simulink model "ADCS_onOrbit"  (R2024b)
settings: Solver=ode4  StartTime=0.0  StopTime=tspan  FixedStep=baseRate  RelTol=1e-3
values from neighbouring files (symbols this model uses):
  A_list = [10*30; 10*30; 10*10; 10*30; 10*30; 10*10] * 1e-04    [adcsInitializer.m]
  A_m = eye(3)    [adcsInitializer.m]
  A_w = eye(3)    [adcsInitializer.m]
  CD = 2.3    [adcsInitializer.m]
  COP = [xAxis/2   0          0 ... (first row only)    [adcsInitializer.m]
  dt = 1    [adcsInitializer.m]
  dYear = decyear(YYYY,MM,DD)    [adcsInitializer.m]
  eta = 0.3    [adcsInitializer.m]
  J_body = [ I_xx  I_xy  I_xz ... (first row only)    [adcsInitializer.m]
  JD0 = juliandate(YYYY,MM,DD,HH,MIN,SEC)    [adcsInitializer.m]
  m = 4    [adcsInitializer.m]
  mag_moment = [0.005; 0.005; 0.005]    [adcsInitializer.m]
  mode = mode(:)    [generateOutput.m]
  mu = 398600.4418    [adcsInitializer.m]    (also in montecarlo.m = mean(W,2))
  n_list = [1 0 0; 0 1 0; 0 0 1; -1 0 0; 0 -1 0; 0 0 -1]    [adcsInitializer.m]
  p = 0.00000451    (= 4.51e-06)    [adcsInitializer.m]
  R = blkdiag(sigma_S^2*eye(3), sigma_B^2*eye(3))    [adcsInitializer.m]
  rE = 6378.14    [adcsInitializer.m]
  sigma_b = deg2rad(0.04)/3600    [adcsInitializer.m]
  sigma_B = 0.001    [adcsInitializer.m]
  sigma_g = deg2rad(0.1)/sqrt(3600)    [adcsInitializer.m]
  sigma_S = deg2rad(0.01)    [adcsInitializer.m]
  T = 1    [adcsInitializer.m]
  wE = [0 0 15.04*(pi/180)*(1/3600)]    [adcsInitializer.m]
  wW_1 = 0    [adcsInitializer.m]
  wW_2 = 0    [adcsInitializer.m]
  wW_3 = 0    [adcsInitializer.m]
undefined symbols (not defined in the file or in its folder): DiscIntNeverNeededParam, J_wheels, K_d, K_p, K_w, n, period, q1_ini, q2_ini, q3_ini, q4_ini, r_I_ini, truevals, useFilter, v_I_ini, wB_1, wB_2, wB_3
libraries: simulink_extras x15, matrix_library x3
(part 1 of 2)
settings Model: Creator=nimis  LastModifiedBy=nimis
settings DebuggingCC: AlgebraicLoopMsg=none

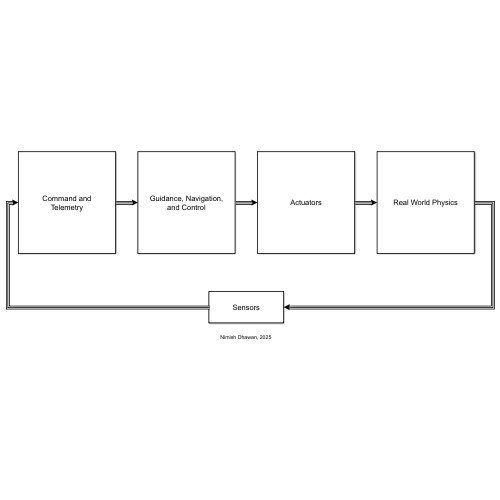
[thumbnail: Simulink's stored preview of the top-level diagram]
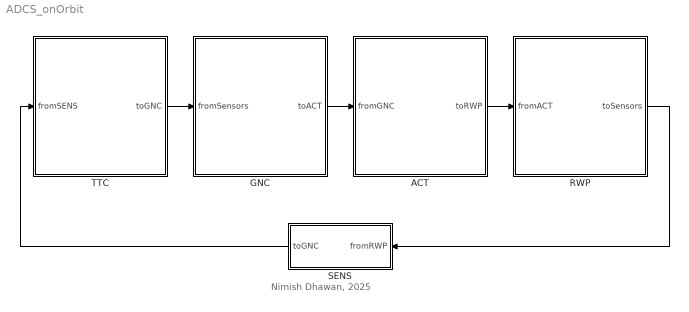
== system ADCS_onOrbit ==
  note: Nimish Dhawan, 2025
  ACT : Subsystem
      mask Display: disp('Actuators');
  GNC : Subsystem
      mask Display: disp('Guidance, Navigation,\nand Control');
  RWP : Subsystem
      mask Display: disp('Real World Physics');
  SENS : Subsystem
      mask Display: disp('Sensors');
  TTC : Subsystem
      mask Display: disp('Command and\nTelemetry');
  wires:
  SENS/1(toGNC) -> TTC/1(fromSENS)
  TTC/1(toGNC) -> GNC/1(fromSensors)
  GNC/1(toACT) -> ACT/1(fromGNC)
  RWP/1(toSensors) -> SENS/1(fromRWP)
  ACT/1(toRWP) -> RWP/1(fromACT)

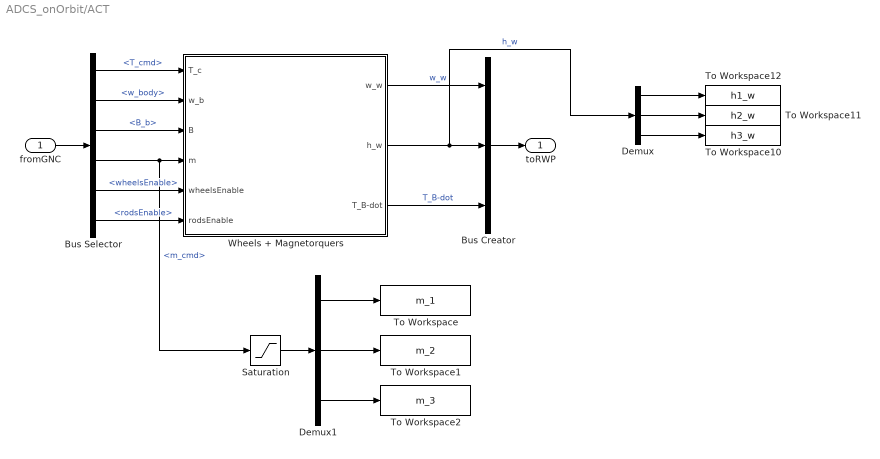
== system ADCS_onOrbit/ACT ==
  fromGNC : Inport
  Bus Creator : BusCreator  Inputs=3
  Bus Selector : BusSelector  OutputSignals=T_cmd,w_body,B_b,m_cmd,wheelsEnable,rodsEnable
  Demux : Demux  Outputs=3
  Demux1 : Demux  Outputs=3
  Saturation : Saturate  UpperLimit=0.2  LowerLimit=-0.2
  To Workspace : ToWorkspace  VariableName=m_1  SampleTime=-1
  To Workspace1 : ToWorkspace  VariableName=m_2  SampleTime=-1
  To Workspace10 : ToWorkspace  VariableName=h3_w  SampleTime=-1
      settings: Save2DSignal=2-D array (concatenate along first dimension)
  To Workspace11 : ToWorkspace  VariableName=h2_w  SampleTime=-1
      settings: Save2DSignal=2-D array (concatenate along first dimension)
  To Workspace12 : ToWorkspace  VariableName=h1_w  SampleTime=-1
      settings: Save2DSignal=2-D array (concatenate along first dimension)
  To Workspace2 : ToWorkspace  VariableName=m_3  SampleTime=-1
  Wheels + Magnetorquers : Subsystem
      mask Display: disp('Wheels + Magnetorquers');
  toRWP : Outport
  wires:
  Bus Selector/2 -> Wheels + Magnetorquers/2(w_b)  "<w_body>"
  Bus Selector/3 -> Wheels + Magnetorquers/3(B)  "<B_b>"
  Bus Selector/4 -> Wheels + Magnetorquers/4(m), Saturation/1  "<m_cmd>"
  Wheels + Magnetorquers/3(T_B-dot) -> Bus Creator/3  "T_B-dot"
  Demux/3 -> To Workspace10/1
  Demux/2 -> To Workspace11/1
  Wheels + Magnetorquers/2(h_w) -> Demux/1, Bus Creator/2  "h_w"
  Demux/1 -> To Workspace12/1
  Demux1/1 -> To Workspace/1
  Saturation/1 -> Demux1/1
  Demux1/2 -> To Workspace1/1
  Demux1/3 -> To Workspace2/1
  fromGNC/1 -> Bus Selector/1
  Bus Selector/1 -> Wheels + Magnetorquers/1(T_c)  "<T_cmd>"
  Bus Creator/1 -> toRWP/1
  Wheels + Magnetorquers/1(w_w) -> Bus Creator/1  "w_w"
  Bus Selector/5 -> Wheels + Magnetorquers/5(wheelsEnable)  "<wheelsEnable>"
  Bus Selector/6 -> Wheels + Magnetorquers/6(rodsEnable)  "<rodsEnable>"

== system ADCS_onOrbit/GNC ==
  fromSensors : Inport
  Bus Creator : BusCreator  Inputs=7
  Bus Selector : BusSelector  OutputSignals=fromSENS,opMode
  Bus Selector1 : BusSelector  OutputSignals=fromSENS.state_act,fromSENS.s_I,opMode
  Bus Selector2 : BusSelector  OutputSignals=fromSENS.h_w,opMode,wheelsEnable,rodsEnable
  Control : Subsystem
  Guidance : Subsystem
      settings: PortSchema="{\"entries\":[{\"content\":{\"sides\":[{\"content\":{},\"type\":\"ConnectorPlacement.EquallySpacedRectSide\",\"uuid\":\"1b864df5-58d8-4c90-91c9-86121554aa4c\"},{\"content\":{\"side\":\"RIGHT\"},\"type\":\"ConnectorPlacement.EquallySpacedRectSide\",\"uuid\":\"8c8748bb-fc8a-40e3-a181-470f6593a9be\"},{\"content\":{\"connectorIds\":[\"Out1\"],\"side\":\"TOP\"},\"type\":\"ConnectorPlacement.EquallySpacedRectSide\",\"uuid\":\"61030da7-ff27-4452-a972-ecb51c641993\"},{\"content\":{\"connectorIds\":[\"In1\",\"In2\",\"In3\",\"In4\",\"In5\"],\"side\":\"BOTTOM\"},\"type\":\"ConnectorPlacement.EquallySpacedRectSide\",\"uuid\":\"02e92b40-894b-4184-ac6b-030597657a3a\"}]},\"type\":\"ConnectorPlacement.EquallySpacedConnector\",\"uuid\":\"ef994289-427e-4085-aff4-2d7817af2aa7\"}],\"packageUris\":[\"http://schema.mathworks.com/mf0/Connector/R2020b\"],\"version\":\"1.0\"}"
  Navigation : Subsystem
  toACT : Outport
  wires:
  Control/4(m) -> Bus Creator/4  "m_cmd"
  Control/2(B_b) -> Bus Creator/2  "B_b"
  Control/1(T_c) -> Bus Creator/1  "T_cmd"
  Bus Selector2/1 -> Control/4(h_w)  "<h_w>"
  Control/3(w_b) -> Bus Creator/3  "w_body"
  fromSensors/1 -> Bus Selector1/1, Bus Selector2/1, Bus Selector/1
  Bus Creator/1 -> toACT/1
  Navigation/1(w_est) -> Control/2(w_body), Guidance/4(w_est)
  Navigation/2(q_est) -> Guidance/5(q_est)  "q_est"
  Navigation/3(B_est) -> Control/3(B)
  Bus Selector1/1 -> Guidance/1(state)  "<state_act>"
  Bus Selector1/2 -> Guidance/2(s_I)  "<s_I>"
  Bus Selector1/3 -> Guidance/3(opMode)  "<opMode>"
  Bus Selector/1 -> Navigation/1(fromSENS)  "<fromSENS>"
  Bus Selector2/2 -> Control/5(opMode), Bus Creator/5  "<opMode>"
  Bus Selector/2 -> Navigation/2(opMode)  "<opMode>"
  Bus Selector2/3 -> Bus Creator/6  "<wheelsEnable>"
  Bus Selector2/4 -> Bus Creator/7  "<rodsEnable>"
  Guidance/1(error) -> Control/1(error)

== system ADCS_onOrbit/RWP ==
  fromACT : Inport
  Environment : Subsystem
  Nonlinear Spacecraft : Subsystem
  Orbit Propator : Subsystem
  Subsystem : Subsystem
  toSensors : Outport
  wires:
  Orbit Propator/1(propOut) -> Environment/1(propIn)
  fromACT/1 -> Nonlinear Spacecraft/2(fromACT)
  Environment/1(envOut) -> Nonlinear Spacecraft/1(T_ext)
  Nonlinear Spacecraft/1(scOut) -> Subsystem/1(fromSC), Orbit Propator/1(q_sc)
  Subsystem/1(RWPoutput) -> toSensors/1

== system ADCS_onOrbit/SENS ==
  fromRWP : Inport
  Bus Creator : BusCreator  Inputs=10
  Bus Selector : BusSelector  OutputSignals=state,B_b,s_B,w_sc
  Bus Selector1 : BusSelector  OutputSignals=h_w,r_SI,q_sc
  Bus Selector2 : BusSelector  OutputSignals=B_I,s_I,T_ext
  GPS : Subsystem
  Gyroscope : Subsystem
  Magnetometer : Subsystem
  Sun Sensor : Subsystem
  toGNC : Outport
  wires:
  fromRWP/1 -> Bus Selector2/1, Bus Selector1/1, Bus Selector/1
  Bus Selector/1 -> GPS/1(state)  "<state>"
  GPS/1(state_act) -> Bus Creator/1  "state_act"
  Bus Selector/2 -> Magnetometer/1(B_b)  "<B_b>"
  Magnetometer/1(B_meas) -> Bus Creator/2  "B_b_meas"
  Bus Selector/3 -> Sun Sensor/1(s_B)  "<s_B>"
  Sun Sensor/1(s_B_meas) -> Bus Creator/3  "s_B_meas"
  Bus Creator/1 -> toGNC/1
  Bus Selector/4 -> Gyroscope/1(w_sc)  "<w_sc>"
  Gyroscope/1(w_meas) -> Bus Creator/4  "w_sc_meas"
  Bus Selector1/3 -> Bus Creator/7  "<q_sc>"
  Bus Selector1/2 -> Bus Creator/6  "<r_SI>"
  Bus Selector1/1 -> Bus Creator/5  "<h_w>"
  Bus Selector2/2 -> Bus Creator/9  "<s_I>"
  Bus Selector2/1 -> Bus Creator/8  "<B_I>"
  Bus Selector2/3 -> Bus Creator/10  "<T_ext>"

== system ADCS_onOrbit/TTC ==
  fromSENS : Inport
  Bus Creator : BusCreator  Inputs=4
  Clock : Clock
  Constant : Constant  Value=mode
  From Spreadsheet : FromSpreadsheet  FileName=controlCommand.xlsx  SheetName=commands  Range=B1:E1000  InterpolationWithinTimeRange=Zero order hold  ExtrapolationAfterLastDataPoint=Hold last value
  MATLAB Function : MATLAB Function  TreatAsAtomicUnit=on
  Mux : Mux  Inputs=3
  RES : Subsystem
      mask Display: disp('Telemetry');
  toGNC : Outport
  tag scope: simTime=global
  wires:
  fromSENS/1 -> Bus Creator/1  "fromSENS"
  Bus Creator/1 -> toGNC/1
  Constant/1 -> MATLAB Function/1(internal)
  From Spreadsheet/1 -> Mux/1  "modeData"
  MATLAB Function/1(mode) -> Bus Creator/2  "opMode"
  From Spreadsheet/3 -> Mux/3  "wheelsData"
  From Spreadsheet/2 -> Mux/2  "rodsData"
  Mux/1 -> MATLAB Function/2(fromTable)
  MATLAB Function/2(wheelsEnable) -> Bus Creator/3  "wheelsEnable"
  MATLAB Function/3(rodsEnable) -> Bus Creator/4  "rodsEnable"
  Clock/1 -> [simTime]

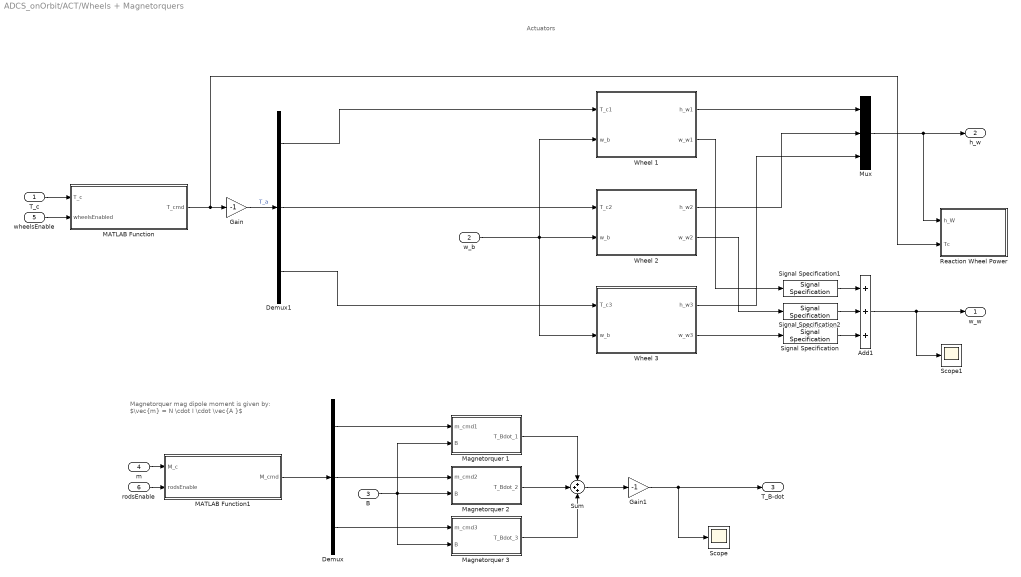
== system ADCS_onOrbit/ACT/Wheels + Magnetorquers ==
  note: Actuators
  note: Magnetorquer mag dipole moment is given by:
      | $\vec{m} = N \cdot I \cdot \vec{A }$
  T_c : Inport
  w_b : Inport  Port=2
  B : Inport  Port=3
  m : Inport  Port=4
  wheelsEnable : Inport  Port=5
  rodsEnable : Inport  Port=6
  Add1 : Sum  Inputs=+++
  Demux : Demux  Outputs=3
  Demux1 : Demux  Outputs=3
  Gain : Gain  Gain=-1
  Gain1 : Gain  Gain=-1
  MATLAB Function : MATLAB Function  TreatAsAtomicUnit=on
  MATLAB Function1 : MATLAB Function  TreatAsAtomicUnit=on
  Magnetorquer 1 : Subsystem
  Magnetorquer 2 : Subsystem
  Magnetorquer 3 : Subsystem
  Mux : Mux  Inputs=3
  Reaction Wheel Power : Subsystem
  Scope : Scope
  Scope1 : Scope
  Signal Specification : SignalSpecification  Dimensions=[3,1]
  Signal Specification1 : SignalSpecification  Dimensions=[3,1]
  Signal Specification2 : SignalSpecification  Dimensions=[3,1]
  Sum : Sum  Inputs=+++
  Wheel 1 : Subsystem
  Wheel 2 : Subsystem
  Wheel 3 : Subsystem
  w_w : Outport
  h_w : Outport  Port=2
  T_B-dot : Outport  Port=3
  wires:
  Gain/1 -> Demux1/1  "T_a"
  T_c/1 -> MATLAB Function/1(T_c)
  Demux1/1 -> Wheel 1/1(T_c1)
  Wheel 3/1(h_w3) -> Mux/3
  Wheel 1/2(w_w1) -> Signal Specification1/1
  w_b/1 -> Wheel 3/2(w_b), Wheel 2/2(w_b), Wheel 1/2(w_b)
  Demux1/2 -> Wheel 2/1(T_c2)
  Mux/1 -> Reaction Wheel Power/1(h_W), h_w/1
  Wheel 1/1(h_w1) -> Mux/1
  Wheel 3/2(w_w3) -> Signal Specification/1
  Demux1/3 -> Wheel 3/1(T_c3)
  Wheel 2/2(w_w2) -> Signal Specification2/1
  Gain1/1 -> T_B-dot/1, Scope/1
  Magnetorquer 3/1(T_Bdot_3) -> Sum/3
  Demux/2 -> Magnetorquer 2/1(m_cmd2)
  Magnetorquer 2/1(T_Bdot_2) -> Sum/2
  Demux/3 -> Magnetorquer 3/1(m_cmd3)
  Sum/1 -> Gain1/1
  Magnetorquer 1/1(T_Bdot_1) -> Sum/1
  B/1 -> Magnetorquer 2/2(B), Magnetorquer 3/2(B), Magnetorquer 1/2(B)
  Demux/1 -> Magnetorquer 1/1(m_cmd1)
  m/1 -> MATLAB Function1/1(M_c)
  Wheel 2/1(h_w2) -> Mux/2
  wheelsEnable/1 -> MATLAB Function/2(wheelsEnabled)
  rodsEnable/1 -> MATLAB Function1/2(rodsEnable)
  MATLAB Function1/1(M_cmd) -> Demux/1
  MATLAB Function/1(T_cmd) -> Reaction Wheel Power/2(Tc), Gain/1
  Add1/1 -> Scope1/1, w_w/1
  Signal Specification/1 -> Add1/3
  Signal Specification1/1 -> Add1/1
  Signal Specification2/1 -> Add1/2

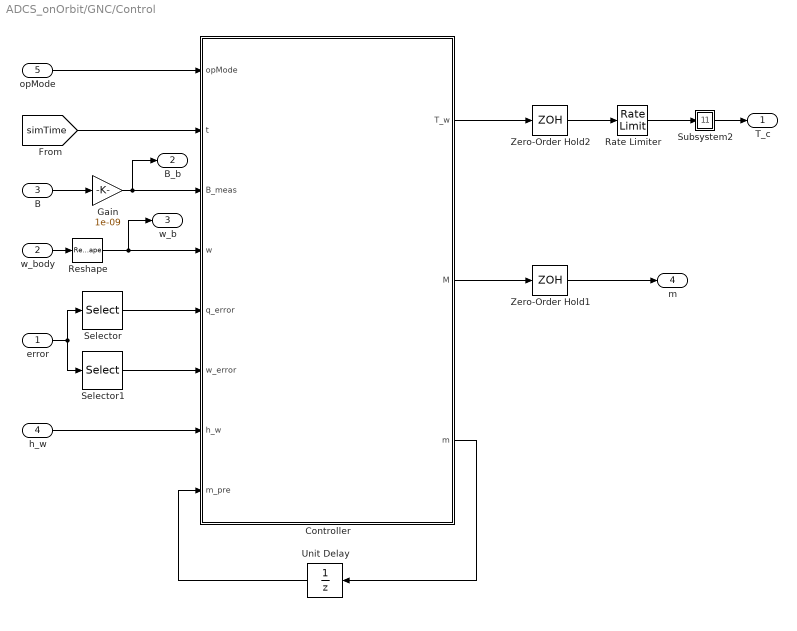
== system ADCS_onOrbit/GNC/Control ==
  error : Inport
  w_body : Inport  Port=2
  B : Inport  Port=3
  h_w : Inport  Port=4
  opMode : Inport  Port=5
  Controller : MATLAB Function  TreatAsAtomicUnit=on
  Gain : Gain  Gain=1e-09
  Rate Limiter : RateLimiter  RisingSlewLimit=5e-07  FallingSlewLimit=-5e-07  SampleTimeMode=inherited
  Reshape : Reshape  OutputDimensionality=Column vector (2-D)  OutputDimensions=[3,1]
  Selector : Selector  InputPortWidth=7  IndexOptions=Index vector (dialog)  Indices=[4 5 6 7]  OutputSizes=1
  Selector1 : Selector  InputPortWidth=7  IndexOptions=Index vector (dialog)  Indices=[1 2 3]  OutputSizes=1
  Subsystem2 : Subsystem
  Unit Delay : UnitDelay  SampleTime=-1  HasFrameUpgradeWarning=on
  Zero-Order Hold1 : ZeroOrderHold  SampleTime=-1
  Zero-Order Hold2 : ZeroOrderHold  SampleTime=-1
  T_c : Outport
  B_b : Outport  Port=2
  w_b : Outport  Port=3
  m : Outport  Port=4
  wires:
  Reshape/1 -> w_b/1, Controller/4(w)
  Gain/1 -> B_b/1, Controller/3(B_meas)
  Controller/1(T_w) -> Zero-Order Hold2/1
  B/1 -> Gain/1
  Zero-Order Hold1/1 -> m/1
  error/1 -> Selector/1, Selector1/1
  Subsystem2/1(T_c) -> T_c/1
  opMode/1 -> Controller/1(opMode)
  [simTime] -> Controller/2(t)
  Selector/1 -> Controller/5(q_error)
  Selector1/1 -> Controller/6(w_error)
  w_body/1 -> Reshape/1
  h_w/1 -> Controller/7(h_w)
  Controller/2(M) -> Zero-Order Hold1/1
  Zero-Order Hold2/1 -> Rate Limiter/1
  Controller/3(m) -> Unit Delay/1
  Unit Delay/1 -> Controller/8(m_pre)
  Rate Limiter/1 -> Subsystem2/1(In1)

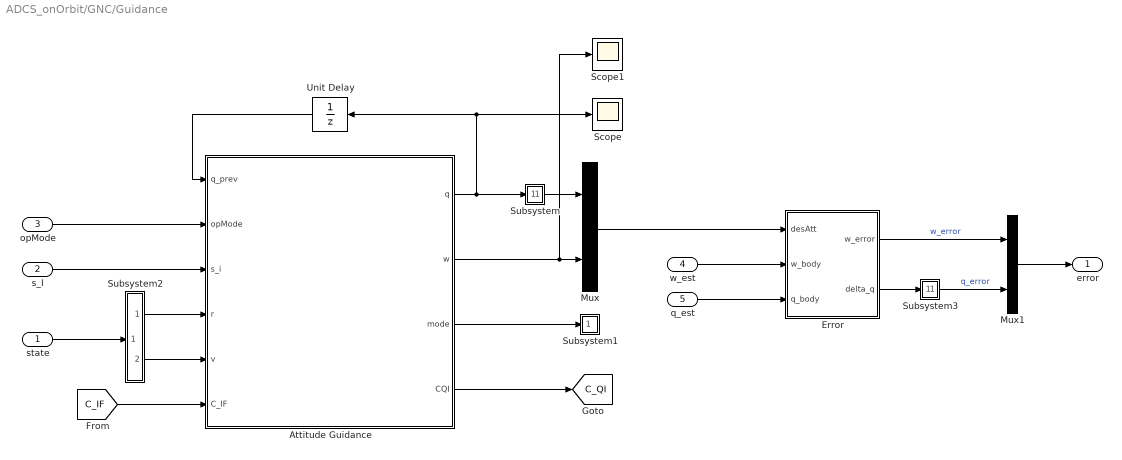
== system ADCS_onOrbit/GNC/Guidance ==
  state : Inport
  s_I : Inport  Port=2
  opMode : Inport  Port=3
  w_est : Inport  Port=4
  q_est : Inport  Port=5
  Attitude Guidance : MATLAB Function  TreatAsAtomicUnit=on
  Error : Subsystem
  Mux : Mux  Inputs=2
  Mux1 : Mux  Inputs=2
  Scope : Scope
  Scope1 : Scope
  Subsystem : Subsystem
  Subsystem1 : Subsystem
  Subsystem2 : Subsystem
      mask Display:
      | port_label('output', 1, 'r');
      | port_label('output', 2, 'v');
  Subsystem3 : Subsystem
  Unit Delay : UnitDelay  InitialCondition=[q1_ini; q2_ini; q3_ini; q4_ini]  SampleTime=-1  HasFrameUpgradeWarning=on
  error : Outport
  tag scope: C_QI=global
  wires:
  Error/2(delta_q) -> Subsystem3/1(q)
  w_est/1 -> Error/2(w_body)
  q_est/1 -> Error/3(q_body)
  Error/1(w_error) -> Mux1/1  "w_error"
  Subsystem3/1(Out1) -> Mux1/2  "q_error"
  Mux1/1 -> error/1
  Subsystem/1(Out1) -> Mux/1
  state/1 -> Subsystem2/1(In1)
  s_I/1 -> Attitude Guidance/3(s_i)
  opMode/1 -> Attitude Guidance/2(opMode)
  Attitude Guidance/1(q) -> Subsystem/1(In1), Scope/1, Unit Delay/1
  Unit Delay/1 -> Attitude Guidance/1(q_prev)
  Subsystem2/1(Out1) -> Attitude Guidance/4(r)
  Subsystem2/2(Out2) -> Attitude Guidance/5(v)
  [C_IF] -> Attitude Guidance/6(C_IF)
  Attitude Guidance/2(w) -> Scope1/1, Mux/2
  Attitude Guidance/3(mode) -> Subsystem1/1(In1)
  Attitude Guidance/4(CQI) -> [C_QI]
  Mux/1 -> Error/1(desAtt)

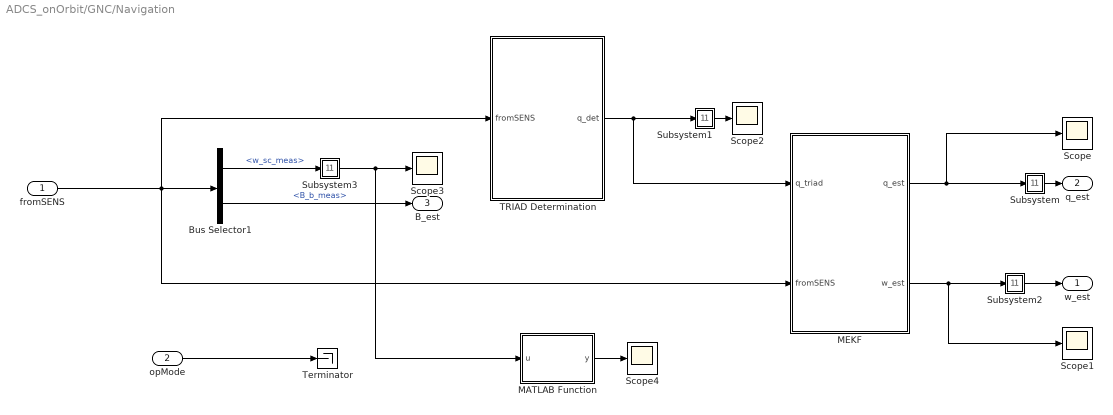
== system ADCS_onOrbit/GNC/Navigation ==
  fromSENS : Inport
  opMode : Inport  Port=2
  Bus Selector1 : BusSelector  OutputSignals=w_sc_meas,B_b_meas
  MATLAB Function : MATLAB Function  TreatAsAtomicUnit=on
  MEKF : Subsystem
  Scope{,1..4} (5 alike) : Scope
  Subsystem : Subsystem
  Subsystem1 : Subsystem
  Subsystem2 : Subsystem
  Subsystem3 : Subsystem
  TRIAD Determination : Subsystem
  Terminator : Terminator
  w_est : Outport
  q_est : Outport  Port=2
  B_est : Outport  Port=3
  wires:
  fromSENS/1 -> MEKF/2(fromSENS), TRIAD Determination/1(fromSENS), Bus Selector1/1
  Bus Selector1/1 -> Subsystem3/1(In1)  "<w_sc_meas>"
  Bus Selector1/2 -> B_est/1  "<B_b_meas>"
  TRIAD Determination/1(q_det) -> Subsystem1/1(q), MEKF/1(q_triad)
  opMode/1 -> Terminator/1
  MEKF/2(w_est) -> Scope1/1, Subsystem2/1(In1)
  MEKF/1(q_est) -> Scope/1, Subsystem/1(q)
  Subsystem2/1(Out1) -> w_est/1
  Subsystem/1(Out1) -> q_est/1
  Subsystem3/1(Out1) -> MATLAB Function/1(u), Scope3/1
  Subsystem1/1(Out1) -> Scope2/1
  MATLAB Function/1(y) -> Scope4/1

== system ADCS_onOrbit/RWP/Environment ==
  propIn : Inport
  Bus Creator : BusCreator  Inputs=5
  Bus Selector : BusSelector  OutputSignals=C_BI,s_I,state
  ENV : Subsystem  VariantControl=ext_torque == true
  MATLAB Function : MATLAB Function  TreatAsAtomicUnit=on
  Scope : Scope
  To Workspace : ToWorkspace  VariableName=T_ext  SampleTime=-1
  envOut : Outport
  wires:
  ENV/3(a_drag) -> Bus Creator/3  "a_drag"
  MATLAB Function/1(y) -> Scope/1, To Workspace/1
  Bus Selector/2 -> ENV/2(s)  "<s_I>"
  Bus Selector/3 -> ENV/3(state)  "<state>"
  ENV/2(T_ext) -> MATLAB Function/1(u), Bus Creator/2  "T_ext"
  ENV/1(B_b) -> Bus Creator/1  "B_b"
  Bus Selector/1 -> ENV/1(C_BI)  "<C_BI>"
  ENV/4(B_I) -> Bus Creator/4  "B_I"
  Bus Creator/1 -> envOut/1
  propIn/1 -> Bus Creator/5, Bus Selector/1  "propOut"

== system ADCS_onOrbit/RWP/Nonlinear Spacecraft ==
  T_ext : Inport
  fromACT : Inport  Port=2
  Bus Creator : BusCreator  Inputs=5
  Bus Selector : BusSelector  OutputSignals=T_ext
  Bus Selector1 : BusSelector  OutputSignals=h_w,T_B-dot
  Scope : Scope
  Spacecraft Dynamics : Subsystem
      settings: PortSchema="{\"entries\":[{\"content\":{\"sides\":[{\"content\":{\"connectorIds\":[\"In1\",\"In2\"]},\"type\":\"ConnectorPlacement.EquallySpacedRectSide\",\"uuid\":\"a70cb8db-1d2e-46b2-94ee-90476f7e1e76\"},{\"content\":{\"connectorIds\":[\"Out1\"],\"side\":\"RIGHT\"},\"type\":\"ConnectorPlacement.EquallySpacedRectSide\",\"uuid\":\"1e67ef54-78b0-4c67-9d63-6ae4863d8fe1\"},{\"content\":{\"connectorIds\":[\"In3\"],\"side\":\"TOP\"},\"type\":\"ConnectorPlacement.EquallySpacedRectSide\",\"uuid\":\"0e387c75-b588-4178-984b-3b9728424b1a\"}]},\"type\":\"ConnectorPlacement.EquallySpacedConnector\",\"uuid\":\"f4277efd-790d-441c-8209-2ef1e3c8f609\"}],\"packageUris\":[\"http://schema.mathworks.com/mf0/Connector/R2020b\"],\"version\":\"1.0\"}"
  Spacecraft Kinematics : Subsystem
  Subsystem : Subsystem
  Subsystem1 : Subsystem
  scOut : Outport
  wires:
  T_ext/1 -> Bus Creator/4, Bus Selector/1  "envOut"
  Bus Selector1/2 -> Spacecraft Dynamics/2(T_Bdot)  "<T_B-dot>"
  fromACT/1 -> Bus Creator/5, Bus Selector1/1  "fromACT"
  Spacecraft Kinematics/1(q) -> Scope/1, Subsystem/1(q)
  Spacecraft Dynamics/1(w_b) -> Spacecraft Kinematics/1(w), Subsystem1/1(In1)  "w_sc"
  Bus Creator/1 -> scOut/1
  Bus Selector/1 -> Spacecraft Dynamics/3(T_b)  "<T_ext>"
  Bus Selector1/1 -> Bus Creator/3, Spacecraft Dynamics/1(h_w)  "<h_w>"
  Subsystem/1(Out1) -> Bus Creator/1  "q_sc"
  Subsystem1/1(Out1) -> Bus Creator/2  "w_sc"

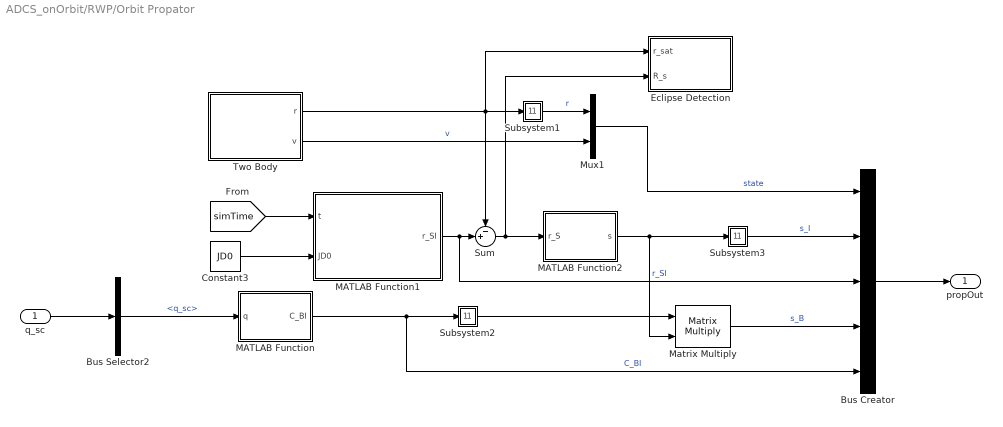
== system ADCS_onOrbit/RWP/Orbit Propator ==
  q_sc : Inport
  Bus Creator : BusCreator  Inputs=5
  Bus Selector2 : BusSelector  OutputSignals=q_sc
  Constant3 : Constant  Value=JD0
  Eclipse Detection : Subsystem
  MATLAB Function : MATLAB Function  TreatAsAtomicUnit=on
  MATLAB Function1 : MATLAB Function  TreatAsAtomicUnit=on
  MATLAB Function2 : MATLAB Function  TreatAsAtomicUnit=on
  Matrix Multiply : Product  Multiplication=Matrix(*)
  Mux1 : Mux  Inputs=2
  Subsystem1 : Subsystem
  Subsystem2 : Subsystem
  Subsystem3 : Subsystem
  Sum : Sum  Inputs=-+|
  Two Body : Subsystem
  propOut : Outport
  wires:
  Bus Creator/1 -> propOut/1
  MATLAB Function/1(C_BI) -> Bus Creator/5, Subsystem2/1(In1)  "C_BI"
  Subsystem3/1(Out1) -> Bus Creator/2  "s_I"
  Subsystem2/1(Out1) -> Matrix Multiply/1
  Subsystem1/1(Out1) -> Mux1/1  "r"
  Bus Selector2/1 -> MATLAB Function/1(q)  "<q_sc>"
  Matrix Multiply/1 -> Bus Creator/4  "s_B"
  MATLAB Function2/1(s) -> Matrix Multiply/2, Subsystem3/1(In1)
  q_sc/1 -> Bus Selector2/1
  Two Body/1(r) -> Eclipse Detection/1(r_sat), Sum/1, Subsystem1/1(In1)
  Two Body/2(v) -> Mux1/2  "v"
  [simTime] -> MATLAB Function1/1(t)
  Constant3/1 -> MATLAB Function1/2(JD0)
  MATLAB Function1/1(r_SI) -> Bus Creator/3, Sum/2  "r_SI"
  Mux1/1 -> Bus Creator/1  "state"
  Sum/1 -> Eclipse Detection/2(R_s), MATLAB Function2/1(r_S)

== system ADCS_onOrbit/RWP/Subsystem ==
  fromSC : Inport
  Bus Creator : BusCreator  Inputs=11
  Bus Selector2 : BusSelector  OutputSignals=q_sc,w_sc,envOut,fromACT.h_w,fromACT.w_w
  Bus Selector3 : BusSelector  OutputSignals=B_I,B_b,T_ext,propOut
  Bus Selector4 : BusSelector  OutputSignals=s_I,state,s_B,r_SI
  Subsystem1 : Subsystem
  Subsystem2 : Subsystem
  RWPoutput : Outport
  wires:
  Subsystem1/1(Out1) -> Bus Creator/11  "w_w"
  Bus Selector4/3 -> Bus Creator/8  "<s_B>"
  Bus Selector3/4 -> Bus Selector4/1  "<propOut>"
  Bus Selector3/2 -> Bus Creator/4  "<B_b>"
  Subsystem2/1(Out1) -> Bus Creator/6  "s_I"
  Bus Selector2/3 -> Bus Selector3/1  "<envOut>"
  Bus Selector4/2 -> Bus Creator/7  "<state>"
  Bus Selector4/4 -> Bus Creator/9  "<r_SI>"
  Bus Selector2/2 -> Bus Creator/2  "<w_sc>"
  Bus Selector4/1 -> Subsystem2/1(In1)  "<s_I>"
  Bus Selector3/1 -> Bus Creator/3  "<B_I>"
  Bus Selector2/1 -> Bus Creator/1  "<q_sc>"
  Bus Creator/1 -> RWPoutput/1
  fromSC/1 -> Bus Selector2/1
  Bus Selector3/3 -> Bus Creator/5  "<T_ext>"
  Bus Selector2/4 -> Bus Creator/10  "<h_w>"
  Bus Selector2/5 -> Subsystem1/1(In1)  "<w_w>"

== system ADCS_onOrbit/SENS/GPS ==
  state : Inport
  state_act : Outport
  wires:
  state/1 -> state_act/1

== system ADCS_onOrbit/SENS/Gyroscope ==
  w_sc : Inport
  Constant : Constant  Value=truevals
  Integrator : Integrator  InitialCondition=0.00000001*ones(3,1)
  MATLAB Function : MATLAB Function  TreatAsAtomicUnit=on
  MATLAB Function1 : MATLAB Function  TreatAsAtomicUnit=on
  MATLAB Function2 : MATLAB Function  TreatAsAtomicUnit=on
  Random Number1 : RandomNumber  Variance=sigma_b^2  SampleTime=1
  Random Number2 : RandomNumber  Variance=sigma_g^2  SampleTime=1
  Scope : Scope
  w_meas : Outport
  wires:
  w_sc/1 -> MATLAB Function2/1(true), MATLAB Function1/1(w_sc)
  MATLAB Function/1(biasDot) -> Integrator/1
  Random Number1/1 -> MATLAB Function/1(noise)
  Integrator/1 -> Scope/1, MATLAB Function1/2(bias)
  Random Number2/1 -> MATLAB Function1/3(noise)
  MATLAB Function1/1(w_meas) -> MATLAB Function2/2(meas)
  MATLAB Function2/1(y) -> w_meas/1
  Constant/1 -> MATLAB Function2/3(set)

== system ADCS_onOrbit/SENS/Magnetometer ==
  B_b : Inport
  Constant : Constant  Value=truevals
  Demux : Demux  Outputs=3
  MATLAB Function : MATLAB Function  TreatAsAtomicUnit=on
  Mux : Mux  Inputs=3
  Random Number : RandomNumber  Variance=sigma_B^2  Seed=123  SampleTime=1
  Random Number1 : RandomNumber  Variance=sigma_B^2  Seed=123  SampleTime=1
  Random Number2 : RandomNumber  Variance=sigma_B^2  Seed=123  SampleTime=1
  Sum : Sum  Inputs=|++
  Sum1 : Sum  Inputs=|++
  Sum2 : Sum  Inputs=|++
  B_meas : Outport
  wires:
  Mux/1 -> MATLAB Function/1(meas)
  Sum2/1 -> Mux/3
  Random Number/1 -> Sum/2
  Random Number1/1 -> Sum1/2
  Demux/3 -> Sum2/1
  Demux/2 -> Sum1/1
  Sum1/1 -> Mux/2
  Demux/1 -> Sum/1
  B_b/1 -> MATLAB Function/2(true), Demux/1
  Sum/1 -> Mux/1
  Random Number2/1 -> Sum2/2
  MATLAB Function/1(y) -> B_meas/1
  Constant/1 -> MATLAB Function/3(set)

== system ADCS_onOrbit/SENS/Sun Sensor ==
  note: This assumes that the sun sensor reference frame coincides
      | with the sc body reference frame
  s_B : Inport
  Constant : Constant  Value=truevals
  Demux : Demux  Outputs=3
  MATLAB Function : MATLAB Function  TreatAsAtomicUnit=on
  Mux : Mux  Inputs=3
  Random Number : RandomNumber  Variance=sigma_S^2  SampleTime=1
  Random Number1 : RandomNumber  Variance=sigma_S^2  SampleTime=1
  Random Number2 : RandomNumber  Variance=sigma_S^2  SampleTime=1
  Sum : Sum  Inputs=|++
  Sum1 : Sum  Inputs=|++
  Sum2 : Sum  Inputs=|++
  s_B_meas : Outport
  wires:
  Demux/1 -> Sum/1
  Random Number/1 -> Sum/2
  Demux/2 -> Sum1/1
  Random Number1/1 -> Sum1/2
  Demux/3 -> Sum2/1
  Random Number2/1 -> Sum2/2
  Sum/1 -> Mux/1
  Sum1/1 -> Mux/2
  Sum2/1 -> Mux/3
  s_B/1 -> MATLAB Function/2(true), Demux/1
  Mux/1 -> MATLAB Function/1(meas)
  MATLAB Function/1(y) -> s_B_meas/1
  Constant/1 -> MATLAB Function/3(set)

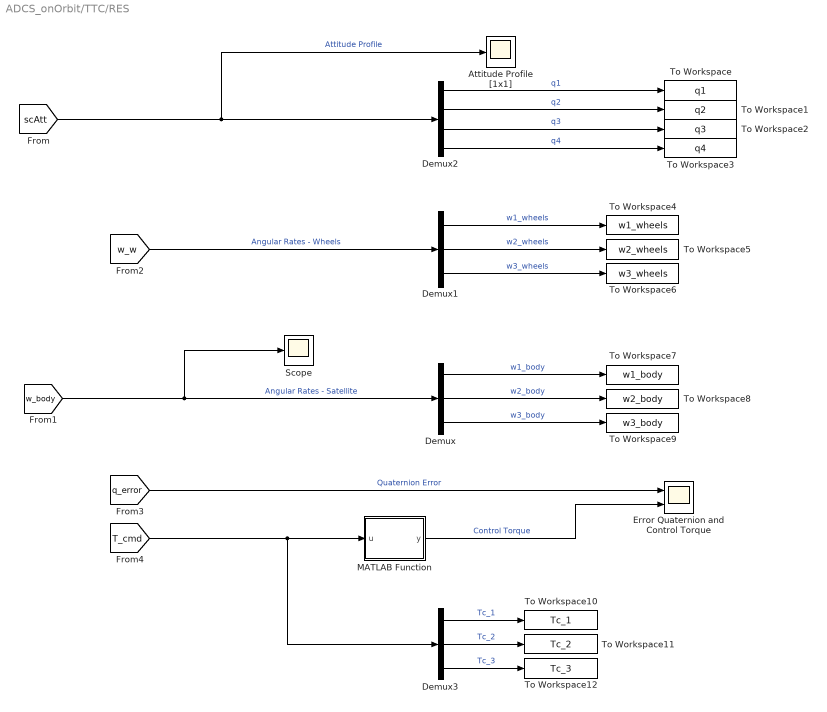
== system ADCS_onOrbit/TTC/RES ==
  Attitude Profile [1x1] : Scope
  Demux : Demux  Outputs=3
  Demux1 : Demux  Outputs=3
  Demux2 : Demux
  Demux3 : Demux  Outputs=3
  Error Quaternion and Control Torque : Scope  NumInputPorts=2
  MATLAB Function : MATLAB Function  TreatAsAtomicUnit=on
  Scope : Scope
  To Workspace : ToWorkspace  VariableName=q1  SampleTime=-1
      settings: Save2DSignal=2-D array (concatenate along first dimension)
  To Workspace1 : ToWorkspace  VariableName=q2  SampleTime=-1
      settings: Save2DSignal=2-D array (concatenate along first dimension)
  To Workspace10 : ToWorkspace  VariableName=Tc_1  SampleTime=-1
      settings: Save2DSignal=2-D array (concatenate along first dimension)
  To Workspace11 : ToWorkspace  VariableName=Tc_2  SampleTime=-1
      settings: Save2DSignal=2-D array (concatenate along first dimension)
  To Workspace12 : ToWorkspace  VariableName=Tc_3  SampleTime=-1
      settings: Save2DSignal=2-D array (concatenate along first dimension)
  To Workspace2 : ToWorkspace  VariableName=q3  SampleTime=-1
      settings: Save2DSignal=2-D array (concatenate along first dimension)
  To Workspace3 : ToWorkspace  VariableName=q4  SampleTime=-1
      settings: Save2DSignal=2-D array (concatenate along first dimension)
  To Workspace4 : ToWorkspace  VariableName=w1_wheels  SampleTime=-1
  To Workspace5 : ToWorkspace  VariableName=w2_wheels  SampleTime=-1
  To Workspace6 : ToWorkspace  VariableName=w3_wheels  SampleTime=-1
  To Workspace7 : ToWorkspace  VariableName=w1_body  SampleTime=-1
  To Workspace8 : ToWorkspace  VariableName=w2_body  SampleTime=-1
  To Workspace9 : ToWorkspace  VariableName=w3_body  SampleTime=-1
  wires:
  Demux1/2 -> To Workspace5/1  "w2_wheels"
  [scAtt] -> Attitude Profile [1x1]/1, Demux2/1  "Attitude Profile"
  Demux/3 -> To Workspace9/1  "w3_body"
  Demux2/3 -> To Workspace2/1  "q3"
  Demux/2 -> To Workspace8/1  "w2_body"
  MATLAB Function/1(y) -> Error Quaternion and Control Torque/2  "Control Torque"
  Demux2/2 -> To Workspace1/1  "q2"
  Demux1/3 -> To Workspace6/1  "w3_wheels"
  Demux2/1 -> To Workspace/1  "q1"
  [w_body] -> Scope/1, Demux/1  "Angular Rates - Satellite"
  Demux1/1 -> To Workspace4/1  "w1_wheels"
  Demux2/4 -> To Workspace3/1  "q4"
  Demux/1 -> To Workspace7/1  "w1_body"
  [T_cmd] -> Demux3/1, MATLAB Function/1(u)
  [w_w] -> Demux1/1  "Angular Rates - Wheels"
  Demux3/1 -> To Workspace10/1  "Tc_1"
  Demux3/2 -> To Workspace11/1  "Tc_2"
  Demux3/3 -> To Workspace12/1  "Tc_3"
  [q_error] -> Error Quaternion and Control Torque/1  "Quaternion Error"

== system ADCS_onOrbit/ACT/Wheels + Magnetorquers/Magnetorquer 1 ==
  m_cmd1 : Inport
  B : Inport  Port=2
  Constant1 : Constant  Value=A_m
  Matrix Multiply : Product
  Matrix Multiply1 : Product  Multiplication=Matrix(*)
  Saturation : Saturate  UpperLimit=0.2  LowerLimit=-0.2
  Submatrix : matrix_library/Submatrix  RowSpan=One row  RowStartMode=Index  RowStartIndex=1  RowEndMode=Last  RowEndIndex=1  ColSpan=All columns  ColStartMode=First  ColStartIndex=1  ColEndMode=Last  ColEndIndex=1
  Transpose : Math  Operator=transpose
  skew symmetric : MATLAB Function  TreatAsAtomicUnit=on
  T_Bdot_1 : Outport
  wires:
  Constant1/1 -> Submatrix/1
  skew symmetric/1(skew) -> Matrix Multiply1/1
  Matrix Multiply1/1 -> T_Bdot_1/1
  Submatrix/1 -> Transpose/1
  Matrix Multiply/1 -> skew symmetric/1(M)
  B/1 -> Matrix Multiply1/2
  Transpose/1 -> Matrix Multiply/2
  m_cmd1/1 -> Saturation/1
  Saturation/1 -> Matrix Multiply/1

== system ADCS_onOrbit/ACT/Wheels + Magnetorquers/Magnetorquer 2 ==
  m_cmd2 : Inport
  B : Inport  Port=2
  Constant1 : Constant  Value=A_m
  Display : Display
  Display1 : Display
  Matrix Multiply : Product
  Matrix Multiply1 : Product  Multiplication=Matrix(*)
  Saturation : Saturate  UpperLimit=0.2  LowerLimit=-0.2
  Submatrix : matrix_library/Submatrix  RowSpan=One row  RowStartMode=Index  RowStartIndex=2  RowEndMode=Last  RowEndIndex=1  ColSpan=All columns  ColStartMode=First  ColStartIndex=1  ColEndMode=Last  ColEndIndex=1
  Transpose : Math  Operator=transpose
  skew symmetric : MATLAB Function  TreatAsAtomicUnit=on
  T_Bdot_2 : Outport
  wires:
  m_cmd2/1 -> Saturation/1
  Transpose/1 -> Matrix Multiply/2
  B/1 -> Matrix Multiply1/2
  Matrix Multiply/1 -> skew symmetric/1(M), Display/1
  Submatrix/1 -> Transpose/1
  Matrix Multiply1/1 -> Display1/1, T_Bdot_2/1
  skew symmetric/1(skew) -> Matrix Multiply1/1
  Constant1/1 -> Submatrix/1
  Saturation/1 -> Matrix Multiply/1

== system ADCS_onOrbit/ACT/Wheels + Magnetorquers/Magnetorquer 3 ==
  m_cmd3 : Inport
  B : Inport  Port=2
  Constant1 : Constant  Value=A_m
  Display : Display
  Display1 : Display
  Matrix Multiply : Product
  Matrix Multiply1 : Product  Multiplication=Matrix(*)
  Saturation : Saturate  UpperLimit=0.2  LowerLimit=-0.2
  Submatrix : matrix_library/Submatrix  RowSpan=One row  RowStartMode=Index  RowStartIndex=3  RowEndMode=Last  RowEndIndex=1  ColSpan=All columns  ColStartMode=First  ColStartIndex=1  ColEndMode=Last  ColEndIndex=1
  Transpose : Math  Operator=transpose
  skew symmetric : MATLAB Function  TreatAsAtomicUnit=on
  T_Bdot_3 : Outport
  wires:
  Constant1/1 -> Submatrix/1
  skew symmetric/1(skew) -> Matrix Multiply1/1
  Matrix Multiply1/1 -> T_Bdot_3/1, Display1/1
  Submatrix/1 -> Transpose/1
  Matrix Multiply/1 -> skew symmetric/1(M), Display/1
  B/1 -> Matrix Multiply1/2
  Transpose/1 -> Matrix Multiply/2
  m_cmd3/1 -> Saturation/1
  Saturation/1 -> Matrix Multiply/1

== system ADCS_onOrbit/ACT/Wheels + Magnetorquers/Reaction Wheel Power ==
  h_W : Inport
  Tc : Inport  Port=2
  MATLAB Function3 : MATLAB Function  TreatAsAtomicUnit=on
  Scope2 : Scope
  Scope4 : Scope
  To Workspace : ToWorkspace  VariableName=Prw  SampleTime=-1
  Unit Delay : UnitDelay  InitialCondition=zeros(3,1)  SampleTime=-1  HasFrameUpgradeWarning=on
  wires:
  MATLAB Function3/1(Prw) -> To Workspace/1, Scope4/1
  Tc/1 -> MATLAB Function3/1(Tc)
  MATLAB Function3/2(Ptotal) -> Unit Delay/1, Scope2/1
  h_W/1 -> MATLAB Function3/2(h_W)
  Unit Delay/1 -> MATLAB Function3/3(P_pre)

== system ADCS_onOrbit/ACT/Wheels + Magnetorquers/Wheel 1 ==
  T_c1 : Inport
  w_b : Inport  Port=2
  Constant1 : Constant  Value=A_w
  Constant2 : Constant  Value=J_wheels
  Integrator1 : Integrator  InitialCondition=wW_1*J_wheels
  MATLAB Function1 : MATLAB Function  TreatAsAtomicUnit=on
  Reshape : Reshape  OutputDimensionality=Column vector (2-D)
  Transfer Fcn : TransferFcn  Numerator=[2.11e04]  Denominator=[J_wheels 1 0]
  Transfer Fcn (with initial states) : simulink_extras/Additional Linear/Transfer Fcn (with initial states)  N=[1]  D="[T  1]"  X0=wW_1*J_wheels
  h_w1 : Outport
  w_w1 : Outport  Port=2
  wires:
  Constant2/1 -> MATLAB Function1/1(J_w)
  T_c1/1 -> Integrator1/1
  w_b/1 -> Reshape/1
  Constant1/1 -> MATLAB Function1/4(A_w)
  MATLAB Function1/1(h_wi) -> h_w1/1
  MATLAB Function1/2(w_wi) -> w_w1/1
  Integrator1/1 -> MATLAB Function1/2(h_w)
  Reshape/1 -> MATLAB Function1/3(wB)

== system ADCS_onOrbit/ACT/Wheels + Magnetorquers/Wheel 2 ==
  T_c2 : Inport
  w_b : Inport  Port=2
  Constant2 : Constant  Value=A_w
  Constant3 : Constant  Value=J_wheels
  Integrator1 : Integrator  InitialCondition=wW_2*J_wheels
  MATLAB Function1 : MATLAB Function  TreatAsAtomicUnit=on
  Reshape : Reshape  OutputDimensionality=Column vector (2-D)
  Transfer Fcn : TransferFcn  Numerator=[2.11e04]  Denominator=[J_wheels 1 0]
  Transfer Fcn (with initial states) : simulink_extras/Additional Linear/Transfer Fcn (with initial states)  N=[1]  D="[T  1]"  X0=wW_2*J_wheels
  h_w2 : Outport
  w_w2 : Outport  Port=2
  wires:
  Constant2/1 -> MATLAB Function1/4(A_w)
  T_c2/1 -> Integrator1/1
  Constant3/1 -> MATLAB Function1/1(J_w)
  MATLAB Function1/2(w_wi) -> w_w2/1
  Integrator1/1 -> MATLAB Function1/2(h_w)
  MATLAB Function1/1(h_wi) -> h_w2/1
  w_b/1 -> Reshape/1
  Reshape/1 -> MATLAB Function1/3(wB)

== system ADCS_onOrbit/ACT/Wheels + Magnetorquers/Wheel 3 ==
  T_c3 : Inport
  w_b : Inport  Port=2
  Constant2 : Constant  Value=A_w
  Constant3 : Constant  Value=J_wheels
  Integrator1 : Integrator  InitialCondition=wW_3*J_wheels
  MATLAB Function1 : MATLAB Function  TreatAsAtomicUnit=on
  Reshape : Reshape  OutputDimensionality=Column vector (2-D)
  Transfer Fcn : TransferFcn  Numerator=[2.11e04]  Denominator=[J_wheels 1 0]
  Transfer Fcn (with initial states) : simulink_extras/Additional Linear/Transfer Fcn (with initial states)  N=[1]  D="[T  1]"  X0=wW_3*J_wheels
  h_w3 : Outport
  w_w3 : Outport  Port=2
  wires:
  Constant2/1 -> MATLAB Function1/4(A_w)
  T_c3/1 -> Integrator1/1
  Constant3/1 -> MATLAB Function1/1(J_w)
  MATLAB Function1/2(w_wi) -> w_w3/1
  Integrator1/1 -> MATLAB Function1/2(h_w)
  MATLAB Function1/1(h_wi) -> h_w3/1
  w_b/1 -> Reshape/1
  Reshape/1 -> MATLAB Function1/3(wB)

== system ADCS_onOrbit/GNC/Control/Subsystem2 ==
  In1 : Inport
  T_c : Outport
  tag scope: T_cmd=global
  wires:
  In1/1 -> T_c/1, [T_cmd]

== system ADCS_onOrbit/GNC/Guidance/Error ==
  desAtt : Inport
  w_body : Inport  Port=2
  q_body : Inport  Port=3
  Error Quaternion : MATLAB Function  TreatAsAtomicUnit=on
  MATLAB Function : MATLAB Function  TreatAsAtomicUnit=on
  Scope : Scope
  Scope1 : Scope
  Selector2 : Selector  InputPortWidth=7  IndexOptions=Index vector (dialog)  Indices=[1 2 3 4]  OutputSizes=1
  Selector3 : Selector  InputPortWidth=7  IndexOptions=Index vector (dialog)  Indices=[5 6 7]  OutputSizes=1
  Sum : Sum  Inputs=|-+
  To Workspace3 : ToWorkspace  VariableName=pointing_err  SampleTime=-1
  w_error : Outport
  delta_q : Outport  Port=2
  wires:
  Selector2/1 -> Error Quaternion/2(q_d)
  q_body/1 -> Error Quaternion/1(q)
  w_body/1 -> Sum/1
  Selector3/1 -> Sum/2
  Sum/1 -> Scope1/1, w_error/1
  MATLAB Function/1(theta_e) -> To Workspace3/1, Scope/1
  desAtt/1 -> Selector3/1, Selector2/1
  Error Quaternion/1(delta_q) -> MATLAB Function/1(q_error), delta_q/1

== system ADCS_onOrbit/GNC/Guidance/Subsystem ==
  In1 : Inport
  Demux2 : Demux
  To Workspace : ToWorkspace  VariableName=q1_des  SampleTime=-1
      settings: Save2DSignal=2-D array (concatenate along first dimension)
  To Workspace1 : ToWorkspace  VariableName=q2_des  SampleTime=-1
      settings: Save2DSignal=2-D array (concatenate along first dimension)
  To Workspace2 : ToWorkspace  VariableName=q3_des  SampleTime=-1
      settings: Save2DSignal=2-D array (concatenate along first dimension)
  To Workspace3 : ToWorkspace  VariableName=q4_des  SampleTime=-1
      settings: Save2DSignal=2-D array (concatenate along first dimension)
  Out1 : Outport
  wires:
  In1/1 -> Demux2/1, Out1/1
  Demux2/1 -> To Workspace/1  "q1_des"
  Demux2/2 -> To Workspace1/1  "q2_des"
  Demux2/3 -> To Workspace2/1  "q3_des"
  Demux2/4 -> To Workspace3/1  "q4_des"

== system ADCS_onOrbit/GNC/Guidance/Subsystem1 ==
  In1 : Inport
  To Workspace4 : ToWorkspace  VariableName=mode  SampleTime=-1
      settings: Save2DSignal=2-D array (concatenate along first dimension)
  wires:
  In1/1 -> To Workspace4/1

== system ADCS_onOrbit/GNC/Guidance/Subsystem2 ==
  In1 : Inport
  Selector1 : Selector  InputPortWidth=6  IndexOptions=Index vector (dialog)  Indices=[1 2 3]  OutputSizes=1
  Selector2 : Selector  InputPortWidth=6  IndexOptions=Index vector (dialog)  Indices=[4 5 6]  OutputSizes=1
  Out1 : Outport
  Out2 : Outport  Port=2
  wires:
  Selector1/1 -> Out1/1
  In1/1 -> Selector2/1, Selector1/1
  Selector2/1 -> Out2/1

== system ADCS_onOrbit/GNC/Guidance/Subsystem3 ==
  q : Inport
  MATLAB Function1 : MATLAB Function  TreatAsAtomicUnit=on
  Radians to Degrees : simulink_extras/Transformations/Radians to Degrees
  Radians to Degrees1 : simulink_extras/Transformations/Radians to Degrees
  Radians to Degrees2 : simulink_extras/Transformations/Radians to Degrees
  To Workspace : ToWorkspace  VariableName=roll_err  SampleTime=-1
  To Workspace1 : ToWorkspace  VariableName=pitch_err  SampleTime=-1
  To Workspace2 : ToWorkspace  VariableName=yaw_err  SampleTime=-1
  Out1 : Outport
  tag scope: q_error=global
  wires:
  Radians to Degrees/1 -> To Workspace/1
  MATLAB Function1/2(pitch) -> Radians to Degrees1/1
  Radians to Degrees1/1 -> To Workspace1/1
  q/1 -> MATLAB Function1/1(q), Out1/1, [q_error]
  Radians to Degrees2/1 -> To Workspace2/1
  MATLAB Function1/1(roll) -> Radians to Degrees/1
  MATLAB Function1/3(yaw) -> Radians to Degrees2/1

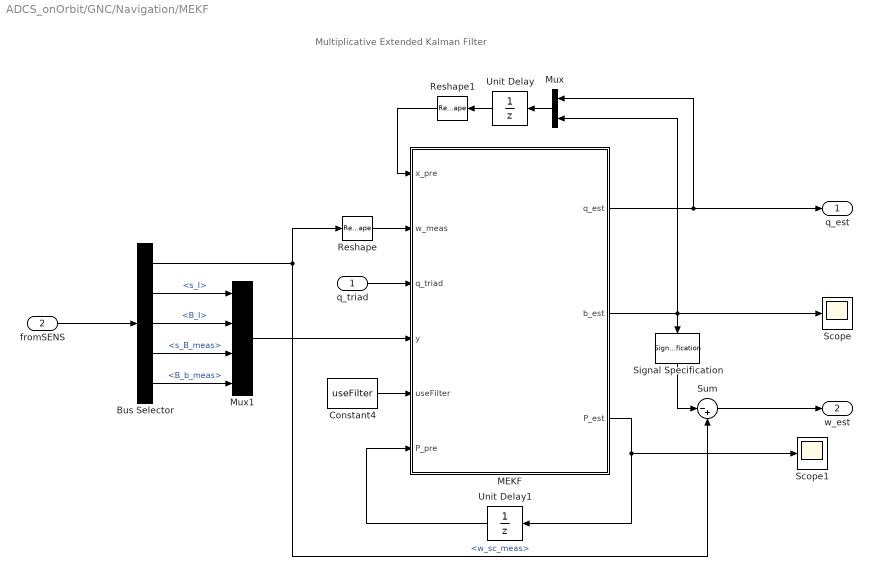
== system ADCS_onOrbit/GNC/Navigation/MEKF ==
  note: Multiplicative Extended Kalman Filter
  q_triad : Inport
  fromSENS : Inport  Port=2
  Bus Selector : BusSelector  OutputSignals=w_sc_meas,s_I,B_I,s_B_meas,B_b_meas
  Constant4 : Constant  Value=useFilter
  MEKF : MATLAB Function  TreatAsAtomicUnit=on
  Mux : Mux  Inputs=2
  Mux1 : Mux
  Reshape : Reshape  OutputDimensionality=Column vector (2-D)
  Reshape1 : Reshape  OutputDimensionality=Customize  OutputDimensions=[7,1]
  Scope : Scope
  Scope1 : Scope
  Signal Specification : SignalSpecification  Dimensions=[3,1]
  Sum : Sum  Inputs=|-+
  Unit Delay : UnitDelay  InitialCondition=[q1_ini; q2_ini; q3_ini; q4_ini; 0.00000001*ones(3,1)]  SampleTime=-1  HasFrameUpgradeWarning=on
  Unit Delay1 : UnitDelay  InitialCondition=0.000001*eye(6)  SampleTime=-1  HasFrameUpgradeWarning=on
  q_est : Outport
  w_est : Outport  Port=2
  wires:
  fromSENS/1 -> Bus Selector/1
  MEKF/3(P_est) -> Unit Delay1/1, Scope1/1
  Unit Delay/1 -> Reshape1/1
  Unit Delay1/1 -> MEKF/6(P_pre)
  Bus Selector/2 -> Mux1/1  "<s_I>"
  Bus Selector/3 -> Mux1/2  "<B_I>"
  Bus Selector/4 -> Mux1/3  "<s_B_meas>"
  Bus Selector/5 -> Mux1/4  "<B_b_meas>"
  Bus Selector/1 -> Sum/2, Reshape/1  "<w_sc_meas>"
  MEKF/1(q_est) -> Mux/1, q_est/1
  MEKF/2(b_est) -> Mux/2, Signal Specification/1, Scope/1
  Sum/1 -> w_est/1
  Mux/1 -> Unit Delay/1
  q_triad/1 -> MEKF/3(q_triad)
  Constant4/1 -> MEKF/5(useFilter)
  Reshape/1 -> MEKF/2(w_meas)
  Reshape1/1 -> MEKF/1(x_pre)
  Mux1/1 -> MEKF/4(y)
  Signal Specification/1 -> Sum/1

== system ADCS_onOrbit/GNC/Navigation/Subsystem ==
  q : Inport
  MATLAB Function2 : MATLAB Function  TreatAsAtomicUnit=on
  Radians to Degrees : simulink_extras/Transformations/Radians to Degrees
  Radians to Degrees1 : simulink_extras/Transformations/Radians to Degrees
  Radians to Degrees2 : simulink_extras/Transformations/Radians to Degrees
  To Workspace : ToWorkspace  VariableName=roll_est  SampleTime=-1
  To Workspace1 : ToWorkspace  VariableName=pitch_est  SampleTime=-1
  To Workspace2 : ToWorkspace  VariableName=yaw_est  SampleTime=-1
  Out1 : Outport
  wires:
  q/1 -> MATLAB Function2/1(q), Out1/1
  Radians to Degrees2/1 -> To Workspace2/1
  Radians to Degrees/1 -> To Workspace/1
  Radians to Degrees1/1 -> To Workspace1/1
  [C_QI] -> MATLAB Function2/2(C_QI)
  MATLAB Function2/1(roll) -> Radians to Degrees/1
  MATLAB Function2/2(pitch) -> Radians to Degrees1/1
  MATLAB Function2/3(yaw) -> Radians to Degrees2/1

== system ADCS_onOrbit/GNC/Navigation/Subsystem1 ==
  q : Inport
  MATLAB Function2 : MATLAB Function  TreatAsAtomicUnit=on
  Radians to Degrees : simulink_extras/Transformations/Radians to Degrees
  Radians to Degrees1 : simulink_extras/Transformations/Radians to Degrees
  Radians to Degrees2 : simulink_extras/Transformations/Radians to Degrees
  To Workspace : ToWorkspace  VariableName=roll_meas  SampleTime=-1
  To Workspace1 : ToWorkspace  VariableName=pitch_meas  SampleTime=-1
  To Workspace2 : ToWorkspace  VariableName=yaw_meas  SampleTime=-1
  Out1 : Outport
  wires:
  MATLAB Function2/3(yaw) -> Radians to Degrees2/1
  MATLAB Function2/2(pitch) -> Radians to Degrees1/1
  MATLAB Function2/1(roll) -> Radians to Degrees/1
  [C_QI] -> MATLAB Function2/2(C_QI)
  Radians to Degrees1/1 -> To Workspace1/1
  Radians to Degrees/1 -> To Workspace/1
  Radians to Degrees2/1 -> To Workspace2/1
  q/1 -> Out1/1, MATLAB Function2/1(q)

== system ADCS_onOrbit/GNC/Navigation/Subsystem2 ==
  In1 : Inport
  Demux : Demux  Outputs=3
  To Workspace : ToWorkspace  VariableName=w1_est  SampleTime=-1
  To Workspace1 : ToWorkspace  VariableName=w2_est  SampleTime=-1
  To Workspace2 : ToWorkspace  VariableName=w3_est  SampleTime=-1
  Out1 : Outport
  wires:
  In1/1 -> Demux/1, Out1/1
  Demux/1 -> To Workspace/1
  Demux/2 -> To Workspace1/1
  Demux/3 -> To Workspace2/1

== system ADCS_onOrbit/GNC/Navigation/Subsystem3 ==
  In1 : Inport
  Demux : Demux  Outputs=3
  To Workspace : ToWorkspace  VariableName=w1_meas  SampleTime=-1
  To Workspace1 : ToWorkspace  VariableName=w2_meas  SampleTime=-1
  To Workspace2 : ToWorkspace  VariableName=w3_meas  SampleTime=-1
  Out1 : Outport
  wires:
  Demux/3 -> To Workspace2/1
  Demux/2 -> To Workspace1/1
  Demux/1 -> To Workspace/1
  In1/1 -> Out1/1, Demux/1

== system ADCS_onOrbit/GNC/Navigation/TRIAD Determination ==
  fromSENS : Inport
  Bus Selector : BusSelector  OutputSignals=s_I,B_I,s_B_meas,B_b_meas
  MATLAB Function1 : MATLAB Function  TreatAsAtomicUnit=on
  Unit Delay : UnitDelay  InitialCondition=[q1_ini; q2_ini; q3_ini; q4_ini]  SampleTime=-1  HasFrameUpgradeWarning=on
  q_det : Outport
  wires:
  Bus Selector/3 -> MATLAB Function1/3(s_b)  "<s_B_meas>"
  Bus Selector/4 -> MATLAB Function1/4(m_b)  "<B_b_meas>"
  fromSENS/1 -> Bus Selector/1
  MATLAB Function1/1(q_triad) -> q_det/1, Unit Delay/1
  Bus Selector/1 -> MATLAB Function1/1(s_I)  "<s_I>"
  Bus Selector/2 -> MATLAB Function1/2(m_I)  "<B_I>"
  Unit Delay/1 -> MATLAB Function1/5(q_prev)

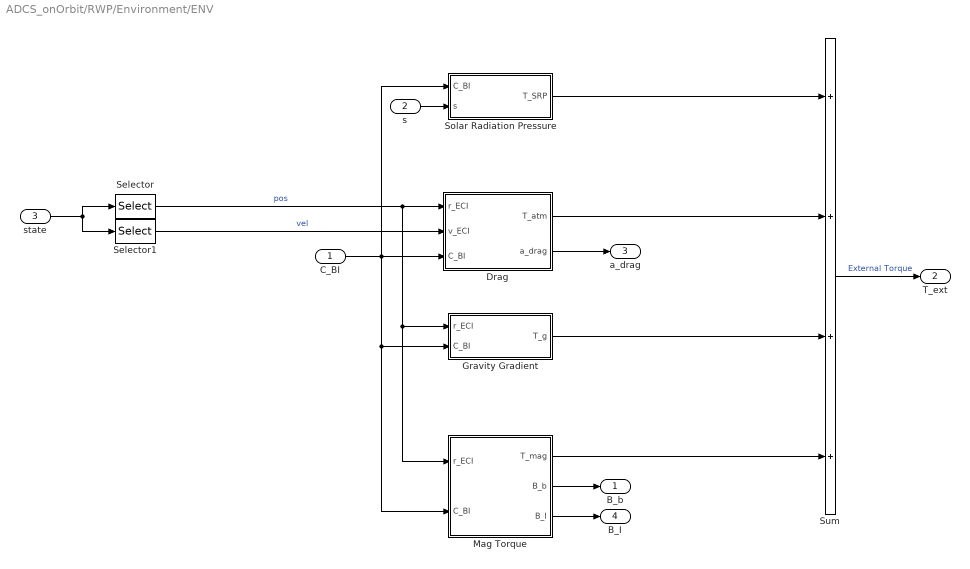
== system ADCS_onOrbit/RWP/Environment/ENV ==
  C_BI : Inport
  s : Inport  Port=2
  state : Inport  Port=3
  Drag : Subsystem
  Gravity Gradient : Subsystem
  Mag Torque : Subsystem
  Selector : Selector  InputPortWidth=6  IndexOptions=Index vector (dialog)  Indices=[1 2 3]  OutputSizes=1
  Selector1 : Selector  InputPortWidth=6  IndexOptions=Index vector (dialog)  Indices=[4 5 6]  OutputSizes=1
  Solar Radiation Pressure : Subsystem
  Sum : Sum  Inputs=++++
  B_b : Outport
  T_ext : Outport  Port=2
  a_drag : Outport  Port=3
  B_I : Outport  Port=4
  wires:
  Drag/2(a_drag) -> a_drag/1
  C_BI/1 -> Solar Radiation Pressure/1(C_BI), Drag/3(C_BI), Gravity Gradient/2(C_BI), Mag Torque/2(C_BI)
  Selector1/1 -> Drag/2(v_ECI)  "vel"
  Gravity Gradient/1(T_g) -> Sum/3
  Sum/1 -> T_ext/1  "External Torque"
  Mag Torque/1(T_mag) -> Sum/4
  Drag/1(T_atm) -> Sum/2
  Selector/1 -> Drag/1(r_ECI), Gravity Gradient/1(r_ECI), Mag Torque/1(r_ECI)  "pos"
  s/1 -> Solar Radiation Pressure/2(s)
  Mag Torque/2(B_b) -> B_b/1
  Solar Radiation Pressure/1(T_SRP) -> Sum/1
  state/1 -> Selector1/1, Selector/1
  Mag Torque/3(B_I) -> B_I/1

== system ADCS_onOrbit/RWP/Nonlinear Spacecraft/Spacecraft Dynamics ==
  h_w : Inport
  T_Bdot : Inport  Port=2
  T_b : Inport  Port=3
  Integrator2 : Integrator  InitialCondition=J_body * [wB_1; wB_2; wB_3]*(pi/180)
  MATLAB Function1 : MATLAB Function  TreatAsAtomicUnit=on
  Reshape : Reshape  OutputDimensionality=Column vector (2-D)  OutputDimensions=[3,1]
  Scope3 : Scope
  Sum2 : Sum
  w_b : Outport
  wires:
  h_w/1 -> Reshape/1
  T_b/1 -> Sum2/1
  T_Bdot/1 -> Sum2/2
  Sum2/1 -> MATLAB Function1/2(T_b)
  Reshape/1 -> MATLAB Function1/3(h_w)
  MATLAB Function1/1(h_tot_dot) -> Integrator2/1
  Integrator2/1 -> MATLAB Function1/1(h_tot)
  MATLAB Function1/2(w_b) -> Scope3/1, w_b/1

== system ADCS_onOrbit/RWP/Nonlinear Spacecraft/Spacecraft Kinematics ==
  note: $\dot \mathbf \epsilon = \frac{1}{2} \left( \eta \ \mathbf I_{3\times3} + \mathbf\epsilon ^{\times} \right) \\ \dot \eta = - \frac{1}{2} \left(\mathbf \epsilon ^{\mathrm{T}} \ \mathbf\omega \right)$
  w : Inport
  Integrator2 : Integrator  InitialCondition=[q1_ini; q2_ini; q3_ini; q4_ini]
  MATLAB Function1 : MATLAB Function  TreatAsAtomicUnit=on
  Quaternion Normalize1 : MATLAB Function  TreatAsAtomicUnit=on
  q : Outport
  wires:
  w/1 -> MATLAB Function1/2(w)
  MATLAB Function1/1(q_dot) -> Integrator2/1
  Integrator2/1 -> Quaternion Normalize1/1(q), MATLAB Function1/1(q)  "q"
  Quaternion Normalize1/1(q_norm) -> q/1

== system ADCS_onOrbit/RWP/Nonlinear Spacecraft/Subsystem ==
  q : Inport
  MATLAB Function2 : MATLAB Function  TreatAsAtomicUnit=on
  Radians to Degrees3 : simulink_extras/Transformations/Radians to Degrees
  Radians to Degrees4 : simulink_extras/Transformations/Radians to Degrees
  Radians to Degrees5 : simulink_extras/Transformations/Radians to Degrees
  To Workspace3 : ToWorkspace  VariableName=roll  SampleTime=-1
  To Workspace4 : ToWorkspace  VariableName=pitch  SampleTime=-1
  To Workspace5 : ToWorkspace  VariableName=yaw  SampleTime=-1
  Out1 : Outport
  tag scope: scAtt=global
  wires:
  Radians to Degrees3/1 -> To Workspace3/1  "roll_deg"
  q/1 -> MATLAB Function2/1(q), Out1/1, [scAtt]
  MATLAB Function2/1(roll) -> Radians to Degrees3/1
  Radians to Degrees5/1 -> To Workspace5/1  "yaw_deg"
  MATLAB Function2/3(yaw) -> Radians to Degrees5/1
  Radians to Degrees4/1 -> To Workspace4/1  "pitch_deg"
  MATLAB Function2/2(pitch) -> Radians to Degrees4/1
  [C_QI] -> MATLAB Function2/2(C_QI)

== system ADCS_onOrbit/RWP/Nonlinear Spacecraft/Subsystem1 ==
  In1 : Inport
  Out1 : Outport
  tag scope: w_body=global
  wires:
  In1/1 -> Out1/1, [w_body]

== system ADCS_onOrbit/RWP/Orbit Propator/Eclipse Detection ==
  r_sat : Inport
  R_s : Inport  Port=2
  Constant1 : Constant  Value=rE
  MATLAB Function3 : MATLAB Function  TreatAsAtomicUnit=on
  Terminator : Terminator
  Unit Delay : UnitDelay  SampleTime=-1  HasFrameUpgradeWarning=on
  tag scope: eclipseExit=global, inEclipse=global
  wires:
  r_sat/1 -> MATLAB Function3/2(r_sat)
  MATLAB Function3/2(eclipse_exit) -> [eclipseExit]
  R_s/1 -> MATLAB Function3/1(R_s)
  Constant1/1 -> MATLAB Function3/3(r_E)
  Unit Delay/1 -> MATLAB Function3/4(was_in_eclipse)
  MATLAB Function3/1(eclipse_entry) -> Terminator/1
  MATLAB Function3/3(is_in_eclipse) -> [inEclipse], Unit Delay/1

== system ADCS_onOrbit/RWP/Orbit Propator/Subsystem1 ==
  In1 : Inport
  Demux : Demux  Outputs=3
  To Workspace1 : ToWorkspace  VariableName=Y_ECI  SampleTime=-1
  To Workspace2 : ToWorkspace  VariableName=Z_ECI  SampleTime=-1
  To Workspace7 : ToWorkspace  VariableName=X_ECI  SampleTime=-1
  Out1 : Outport
  wires:
  In1/1 -> Out1/1, Demux/1
  Demux/1 -> To Workspace7/1
  Demux/2 -> To Workspace1/1
  Demux/3 -> To Workspace2/1

== system ADCS_onOrbit/RWP/Orbit Propator/Subsystem2 ==
  In1 : Inport
  Out1 : Outport
  tag scope: C_BI=global
  wires:
  In1/1 -> [C_BI], Out1/1

== system ADCS_onOrbit/RWP/Orbit Propator/Subsystem3 ==
  In1 : Inport
  Demux : Demux  Outputs=3
  To Workspace1 : ToWorkspace  VariableName=s_y  SampleTime=-1
  To Workspace2 : ToWorkspace  VariableName=s_z  SampleTime=-1
  To Workspace7 : ToWorkspace  VariableName=s_x  SampleTime=-1
  Out1 : Outport
  wires:
  In1/1 -> Out1/1, Demux/1
  Demux/1 -> To Workspace7/1
  Demux/2 -> To Workspace1/1
  Demux/3 -> To Workspace2/1

== system ADCS_onOrbit/RWP/Orbit Propator/Two Body ==
  Constant : Constant  Value=mu
  Constant1 : Constant  Value=rE
  Discrete-Time Integrator : DiscreteIntegrator  Commented=on  gainval=1  InitialCondition=v_I_ini  SampleTime=-1  ICPrevOutput=DiscIntNeverNeededParam  ICPrevScaledInput=DiscIntNeverNeededParam
  Discrete-Time Integrator1 : DiscreteIntegrator  Commented=on  gainval=1  InitialCondition=r_I_ini  SampleTime=-1  ICPrevOutput=DiscIntNeverNeededParam  ICPrevScaledInput=DiscIntNeverNeededParam
  Integrator : Integrator  InitialCondition=v_I_ini
  Integrator1 : Integrator  InitialCondition=r_I_ini
  MATLAB Function1 : MATLAB Function  TreatAsAtomicUnit=on
  MATLAB Function3 : MATLAB Function  TreatAsAtomicUnit=on
  Sum1 : Sum  Inputs=|++
  r : Outport
  v : Outport  Port=2
  wires:
  Constant/1 -> MATLAB Function3/2(mu), MATLAB Function1/2(mu)
  Integrator/1 -> Integrator1/1, v/1
  MATLAB Function3/1(a_j2) -> Sum1/2  "a_J2"
  MATLAB Function1/1(a_I) -> Sum1/1
  Sum1/1 -> Integrator/1
  Integrator1/1 -> r/1, MATLAB Function1/1(r_I), MATLAB Function3/1(r)  "r"
  Constant1/1 -> MATLAB Function3/3(rE)

== system ADCS_onOrbit/RWP/Subsystem/Subsystem1 ==
  In1 : Inport
  Out1 : Outport
  tag scope: w_w=global
  wires:
  In1/1 -> Out1/1, [w_w]

== system ADCS_onOrbit/RWP/Subsystem/Subsystem2 ==
  In1 : Inport
  Out1 : Outport
  tag scope: s_I=global
  wires:
  In1/1 -> [s_I], Out1/1

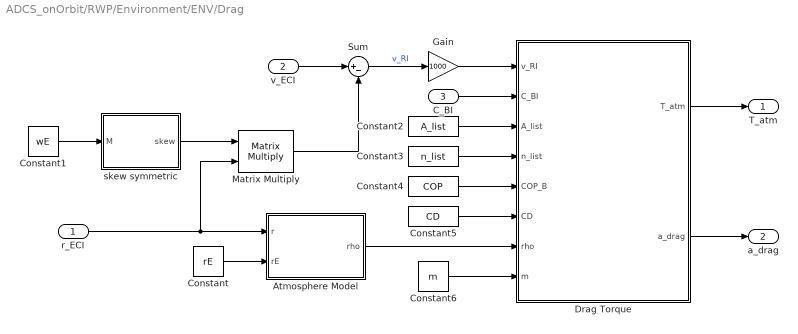
== system ADCS_onOrbit/RWP/Environment/ENV/Drag ==
  r_ECI : Inport
  v_ECI : Inport  Port=2
  C_BI : Inport  Port=3
  Atmosphere Model : MATLAB Function  TreatAsAtomicUnit=on
  Constant : Constant  Value=rE
  Constant1 : Constant  Value=wE
  Constant2 : Constant  Value=A_list
  Constant3 : Constant  Value=n_list
  Constant4 : Constant  Value=COP
  Constant5 : Constant  Value=CD
  Constant6 : Constant  Value=m
  Drag Torque : MATLAB Function  TreatAsAtomicUnit=on
  Gain : Gain  Gain=1000
  Matrix Multiply : Product  Multiplication=Matrix(*)
  Sum : Sum  Inputs=|+-
  skew symmetric : MATLAB Function  TreatAsAtomicUnit=on
  T_atm : Outport
  a_drag : Outport  Port=2
  wires:
  Drag Torque/2(a_drag) -> a_drag/1
  Constant6/1 -> Drag Torque/8(m)
  Atmosphere Model/1(rho) -> Drag Torque/7(rho)
  Constant5/1 -> Drag Torque/6(CD)
  Constant4/1 -> Drag Torque/5(COP_B)
  Constant3/1 -> Drag Torque/4(n_list)
  Constant2/1 -> Drag Torque/3(A_list)
  C_BI/1 -> Drag Torque/2(C_BI)
  Gain/1 -> Drag Torque/1(v_RI)
  Sum/1 -> Gain/1  "v_RI"
  v_ECI/1 -> Sum/1
  Matrix Multiply/1 -> Sum/2
  Drag Torque/1(T_atm) -> T_atm/1
  skew symmetric/1(skew) -> Matrix Multiply/1
  Constant1/1 -> skew symmetric/1(M)
  Constant/1 -> Atmosphere Model/2(rE)
  r_ECI/1 -> Atmosphere Model/1(r), Matrix Multiply/2

== system ADCS_onOrbit/RWP/Environment/ENV/Gravity Gradient ==
  r_ECI : Inport
  C_BI : Inport  Port=2
  Constant : Constant  Value=J_body
  Constant1 : Constant  Value=mu
  MATLAB Function3 : MATLAB Function  TreatAsAtomicUnit=on
  T_g : Outport
  wires:
  C_BI/1 -> MATLAB Function3/4(C_BI)
  Constant/1 -> MATLAB Function3/2(J)
  r_ECI/1 -> MATLAB Function3/1(r_I)
  Constant1/1 -> MATLAB Function3/3(mu)
  MATLAB Function3/1(T_g) -> T_g/1
